simulink model "Control"  (R2020b)
settings: Solver=VariableStepAuto  StartTime=0.0  StopTime=120  RelTol=1e-3
values from neighbouring files (symbols this model uses):
  b = 50.0    [Data.sldd]
  m = 1000.0    [Data.sldd]
settings Model: DataDictionary=Data.sldd  OrderedModelArguments=off  Creator=smart  LastModifiedBy=smart

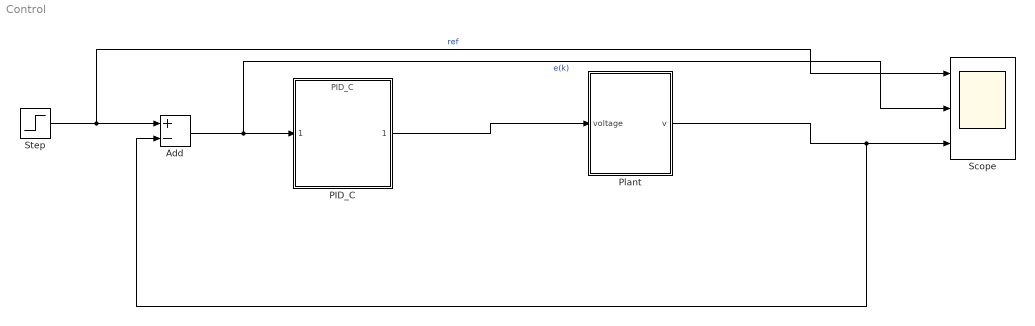
== system Control ==
  Add : Sum  Inputs=+-
  PID_C : ModelReference  ModelNameDialog=PID_C  SimulationMode=Normal  ModelReferenceVersion=1.4
  Plant : Subsystem
  Scope : Scope  NumInputPorts=3
  Step : Step  Time=0  After=500  SampleTime=0
  wires:
  Step/1 -> Scope/1, Add/1  "ref"
  Add/1 -> Scope/2, PID_C/1  "e(k)"
  PID_C/1 -> Plant/1(voltage)
  Plant/1(v) -> Add/2, Scope/3

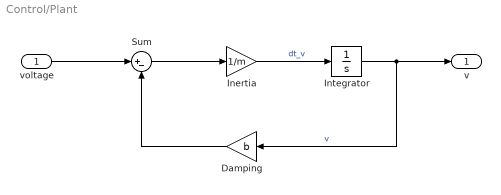
== system Control/Plant ==
  voltage : Inport
  Damping : Gain  Gain=b
  Inertia : Gain  Gain=1/m
  Integrator : Integrator
  Sum : Sum  Inputs=|+-
  v : Outport
  wires:
  Integrator/1 -> v/1, Damping/1  "v"
  Sum/1 -> Inertia/1
  voltage/1 -> Sum/1
  Damping/1 -> Sum/2
  Inertia/1 -> Integrator/1  "dt_v"
